simulink model "sim_on_off"  (R2024b)
settings: Solver=ode45  StartTime=t_0  StopTime=100  FixedStep=dt  RelTol=1e-4
undefined symbols (not defined in the file or in its folder): brake_off, brake_on, const_brake
libraries: simulink x1
settings Model: Creator=yevge  LastModifiedBy=yevge
settings DebuggingCC: AlgebraicLoopMsg=error  CheckMatrixSingularityMsg=error

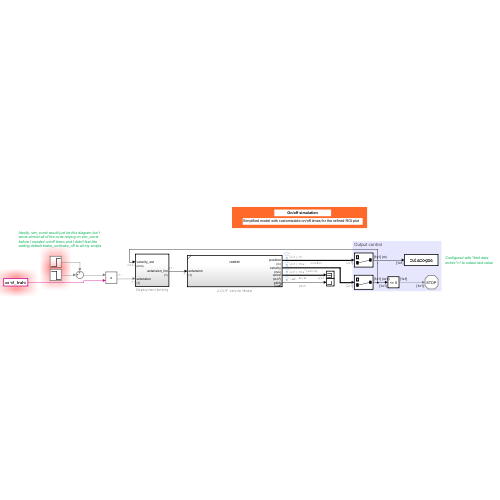
[thumbnail: Simulink's stored preview of the top-level diagram]
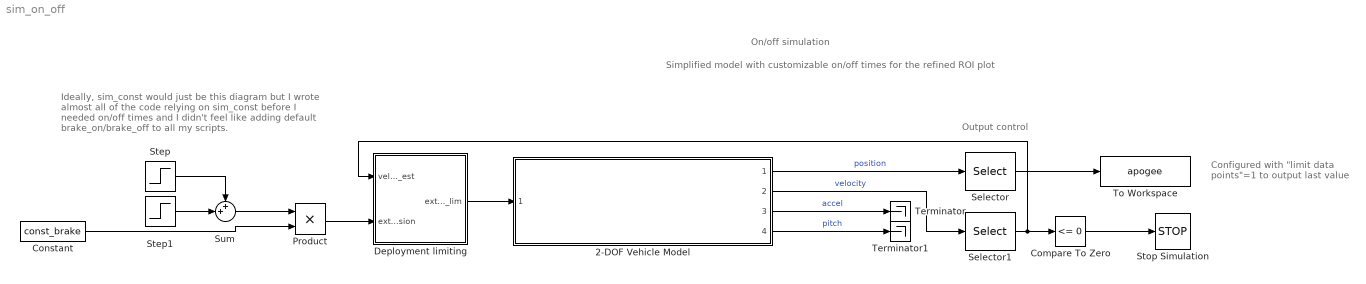
== system sim_on_off ==
  note: Simplified model with customizable on/off times for the refined ROI plot
  note: Configured with "limit data points"=1 to output last value
  note: On/off simulation
  note: Output control
  note: Ideally, sim_const would just be this diagram but I wrote almost all of the code relying on sim_const before I needed on/off times and I didn't feel like adding default brake_on/brake_off to all my scripts.
  2-DOF Vehicle Model : Subsystem  ReferencedSubsystem=rocket
  Compare To Zero : simulink/Logic and Bit Operations/Compare To Zero  relop=<=  OutDataTypeStr=boolean
  Constant : Constant  Value=const_brake
  Deployment limiting : Subsystem
  Product : Product
  Selector : Selector  InputPortWidth=2  IndexOptions=Index vector (dialog)  Indices=2  OutputSizes=1
  Selector1 : Selector  InputPortWidth=2  IndexOptions=Index vector (dialog)  Indices=2  OutputSizes=1
  Step : Step  Time=brake_on  SampleTime=0
  Step1 : Step  Time=brake_off  After=-1  SampleTime=0
  Stop Simulation : Stop
  Sum : Sum  Inputs=++|
  Terminator : Terminator
  Terminator1 : Terminator
  To Workspace : ToWorkspace  VariableName=apogee  SampleTime=-1
      settings: MaxDataPoints=1
  wires:
  Selector/1 -> To Workspace/1
  Selector1/1 -> Deployment limiting/1(velocity_est), Compare To Zero/1
  Compare To Zero/1 -> Stop Simulation/1
  Product/1 -> Deployment limiting/2(extension)
  Deployment limiting/1(extension_lim) -> 2-DOF Vehicle Model/1
  2-DOF Vehicle Model/1 -> Selector/1  "position"
  2-DOF Vehicle Model/3 -> Terminator/1  "accel"
  2-DOF Vehicle Model/2 -> Selector1/1  "velocity"
  2-DOF Vehicle Model/4 -> Terminator1/1  "pitch"
  Step1/1 -> Sum/2
  Step/1 -> Sum/1
  Sum/1 -> Product/1
  Constant/1 -> Product/2

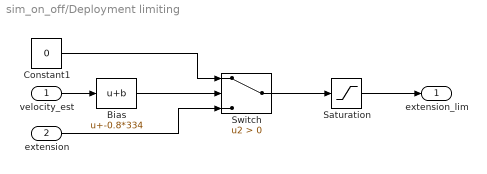
== system sim_on_off/Deployment limiting ==
  velocity_est : Inport  Unit=m/s  PortDimensions=1
  extension : Inport  Port=2  OutMin=0  OutMax=1  Unit=1  PortDimensions=1
  Bias : Bias  Bias=-0.8*334  SaturateOnIntegerOverflow=off
  Constant1 : Constant  Value=0
  Saturation : Saturate  UpperLimit=1  LowerLimit=0
  Switch : Switch  Criteria=u2 > Threshold  SaturateOnIntegerOverflow=off  InputSameDT=off
  extension_lim : Outport  OutMin=0  OutMax=1  Unit=1  PortDimensions=1
  wires:
  Switch/1 -> Saturation/1
  Constant1/1 -> Switch/1
  extension/1 -> Switch/3
  velocity_est/1 -> Bias/1
  Bias/1 -> Switch/2
  Saturation/1 -> extension_lim/1
